simulink model "ctrlAllocMatrix_th"  (R2018b)
settings: Solver=FixedStepDiscrete  StartTime=0.0  StopTime=timeVec(end)  FixedStep=1  RelTol=1e-3
values from neighbouring files (symbols this model uses):
  angVelBdy = [0 0 0]*pi/180    [ctrlAllocMatrix_ts.m]
  velCMBdy = [0 0 0]    [ctrlAllocMatrix_ts.m]
undefined symbols (not defined in the file or in its folder): vhcl
libraries: fluidDynamicSurface_cl x4, ctrlAllocMatrix_cl x1
settings Model: Creator=mcobb  LastModifiedBy=mcobb

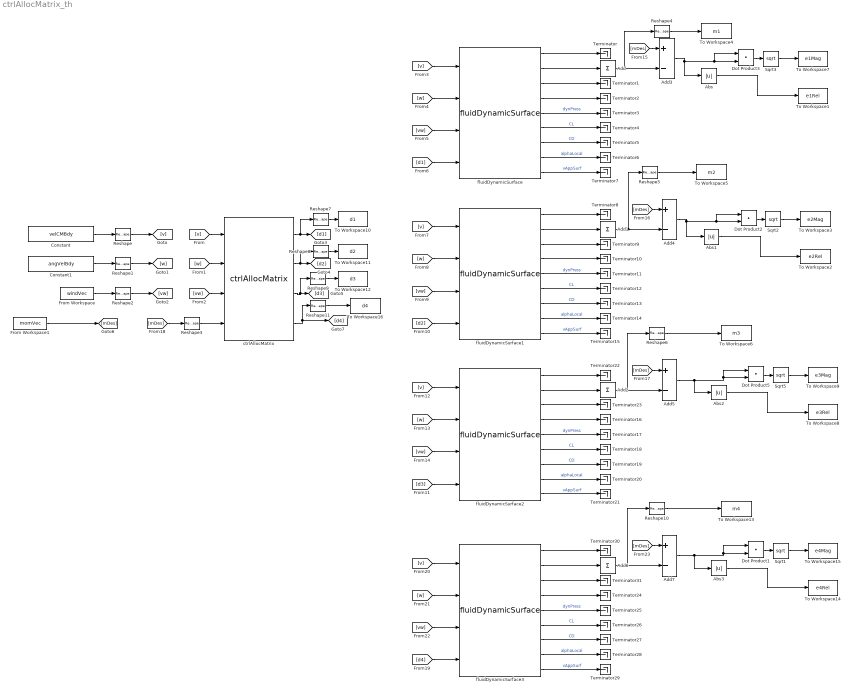
== system ctrlAllocMatrix_th ==
  Abs{,1..3} (4 alike) : Abs
  Add{,1..2,6} (4 alike) : Sum  Inputs=1  CollapseMode=Specified dimension  CollapseDim=2
  Add{3..5,7} (4 alike) : Sum  Inputs=+-
  Constant : Constant  Value=velCMBdy
  Constant1 : Constant  Value=angVelBdy
  Dot Product{1..3,5} (4 alike) : DotProduct  InputSameDT=on  OutDataTypeStr=Inherit: Inherit via internal rule
  From Workspace : FromWorkspace  VariableName=windVec  SampleTime=0
  From Workspace1 : FromWorkspace  VariableName=momVec  SampleTime=0
  Reshape{,1..3} (4 alike) : Reshape  OutputDimensionality=Column vector (2-D)
  Reshape{4..11} (8 alike) : Reshape
  Sqrt{1..3,5} (4 alike) : Sqrt  SaturateOnIntegerOverflow=on
  Terminator{,1..31} (32 alike) : Terminator
  To Workspace1 : ToWorkspace  VariableName=e1Rel  SaveFormat=Timeseries  SampleTime=-1
  To Workspace10 : ToWorkspace  VariableName=d1  SaveFormat=Timeseries  SampleTime=-1
  To Workspace11 : ToWorkspace  VariableName=d2  SaveFormat=Timeseries  SampleTime=-1
  To Workspace12 : ToWorkspace  VariableName=d3  SaveFormat=Timeseries  SampleTime=-1
  To Workspace13 : ToWorkspace  VariableName=m4  SaveFormat=Timeseries  SampleTime=-1
  To Workspace14 : ToWorkspace  VariableName=e4Rel  SaveFormat=Timeseries  SampleTime=-1
  To Workspace15 : ToWorkspace  VariableName=e4Mag  SaveFormat=Timeseries  SampleTime=-1
  To Workspace16 : ToWorkspace  VariableName=d4  SaveFormat=Timeseries  SampleTime=-1
  To Workspace2 : ToWorkspace  VariableName=e2Rel  SaveFormat=Timeseries  SampleTime=-1
  To Workspace3 : ToWorkspace  VariableName=e2Mag  SaveFormat=Timeseries  SampleTime=-1
  To Workspace4 : ToWorkspace  VariableName=m1  SaveFormat=Timeseries  SampleTime=-1
  To Workspace5 : ToWorkspace  VariableName=m2  SaveFormat=Timeseries  SampleTime=-1
  To Workspace6 : ToWorkspace  VariableName=m3  SaveFormat=Timeseries  SampleTime=-1
  To Workspace7 : ToWorkspace  VariableName=e1Mag  SaveFormat=Timeseries  SampleTime=-1
  To Workspace8 : ToWorkspace  VariableName=e3Rel  SaveFormat=Timeseries  SampleTime=-1
  To Workspace9 : ToWorkspace  VariableName=e3Mag  SaveFormat=Timeseries  SampleTime=-1
  ctrlAllocMatrix : ctrlAllocMatrix_cl/ctrlAllocMatrix  aeroStruct=vhcl.struct('OCT.aeroSurf')  fluidDensity=1000  ctrlUpMax=30  ctrlDnMax=-30
  fluidDynamicSurface{,1..3} (4 alike) : fluidDynamicSurface_cl/fluidDynamicSurface  aeroStruct=vhcl.struct('OCT.aeroSurf')  fluidDensity=1000
  wires:
  Constant/1 -> Reshape/1
  Constant1/1 -> Reshape1/1
  From Workspace/1 -> Reshape2/1
  From Workspace1/1 -> [mDes]
  Reshape3/1 -> ctrlAllocMatrix/4
  Reshape/1 -> [v]
  [v] -> ctrlAllocMatrix/1
  [w] -> ctrlAllocMatrix/2
  Reshape1/1 -> [w]
  Reshape2/1 -> [vw]
  [vw] -> ctrlAllocMatrix/3
  [v] -> fluidDynamicSurface/1
  [w] -> fluidDynamicSurface/2
  [vw] -> fluidDynamicSurface/3
  fluidDynamicSurface/1 -> Terminator/1
  fluidDynamicSurface/2 -> Add/1
  fluidDynamicSurface/3 -> Terminator1/1
  fluidDynamicSurface/4 -> Terminator2/1
  fluidDynamicSurface/5 -> Terminator3/1  "dynPress"
  fluidDynamicSurface/6 -> Terminator4/1  "CL"
  fluidDynamicSurface/7 -> Terminator5/1  "CD"
  fluidDynamicSurface/8 -> Terminator6/1  "alphaLocal"
  fluidDynamicSurface/9 -> Terminator7/1  "vAppSurf"
  Add/1 -> Reshape4/1, Add3/2
  ctrlAllocMatrix/1 -> Reshape7/1, [d1]
  ctrlAllocMatrix/2 -> Reshape8/1, [d2]
  ctrlAllocMatrix/3 -> Reshape9/1, [d3]
  [d1] -> fluidDynamicSurface/4
  [d2] -> fluidDynamicSurface1/4
  fluidDynamicSurface1/9 -> Terminator15/1  "vAppSurf"
  fluidDynamicSurface1/8 -> Terminator14/1  "alphaLocal"
  fluidDynamicSurface1/7 -> Terminator13/1  "CD"
  fluidDynamicSurface1/6 -> Terminator12/1  "CL"
  fluidDynamicSurface1/5 -> Terminator11/1  "dynPress"
  fluidDynamicSurface1/4 -> Terminator10/1
  fluidDynamicSurface1/3 -> Terminator9/1
  fluidDynamicSurface1/2 -> Add1/1
  fluidDynamicSurface1/1 -> Terminator8/1
  [vw] -> fluidDynamicSurface1/3
  [w] -> fluidDynamicSurface1/2
  [v] -> fluidDynamicSurface1/1
  [v] -> fluidDynamicSurface2/1
  [w] -> fluidDynamicSurface2/2
  [vw] -> fluidDynamicSurface2/3
  fluidDynamicSurface2/1 -> Terminator22/1
  fluidDynamicSurface2/2 -> Add2/1
  fluidDynamicSurface2/3 -> Terminator23/1
  fluidDynamicSurface2/4 -> Terminator16/1
  fluidDynamicSurface2/5 -> Terminator17/1  "dynPress"
  fluidDynamicSurface2/6 -> Terminator18/1  "CL"
  fluidDynamicSurface2/7 -> Terminator19/1  "CD"
  fluidDynamicSurface2/8 -> Terminator20/1  "alphaLocal"
  fluidDynamicSurface2/9 -> Terminator21/1  "vAppSurf"
  [d3] -> fluidDynamicSurface2/4
  [mDes] -> Add3/1
  Add3/1 -> Dot Product3/1, Dot Product3/2, Abs/1
  [mDes] -> Add4/1
  Add1/1 -> Reshape5/1, Add4/2
  Add2/1 -> Reshape6/1, Add5/2
  [mDes] -> Add5/1
  [mDes] -> Reshape3/1
  Abs/1 -> To Workspace1/1
  Reshape4/1 -> To Workspace4/1
  Reshape5/1 -> To Workspace5/1
  Reshape6/1 -> To Workspace6/1
  Dot Product3/1 -> Sqrt3/1
  Sqrt3/1 -> To Workspace7/1
  Sqrt2/1 -> To Workspace3/1
  Dot Product2/1 -> Sqrt2/1
  Abs1/1 -> To Workspace2/1
  Add4/1 -> Abs1/1, Dot Product2/2, Dot Product2/1
  Add5/1 -> Dot Product5/1, Dot Product5/2, Abs2/1
  Abs2/1 -> To Workspace8/1
  Dot Product5/1 -> Sqrt5/1
  Sqrt5/1 -> To Workspace9/1
  Reshape7/1 -> To Workspace10/1
  Reshape8/1 -> To Workspace11/1
  Reshape9/1 -> To Workspace12/1
  Sqrt1/1 -> To Workspace15/1
  Dot Product1/1 -> Sqrt1/1
  Abs3/1 -> To Workspace14/1
  Add7/1 -> Abs3/1, Dot Product1/2, Dot Product1/1
  Reshape10/1 -> To Workspace13/1
  [mDes] -> Add7/1
  Add6/1 -> Add7/2, Reshape10/1
  [d4] -> fluidDynamicSurface3/4
  fluidDynamicSurface3/9 -> Terminator29/1  "vAppSurf"
  fluidDynamicSurface3/8 -> Terminator28/1  "alphaLocal"
  fluidDynamicSurface3/7 -> Terminator27/1  "CD"
  fluidDynamicSurface3/6 -> Terminator26/1  "CL"
  fluidDynamicSurface3/5 -> Terminator25/1  "dynPress"
  fluidDynamicSurface3/4 -> Terminator24/1
  fluidDynamicSurface3/3 -> Terminator31/1
  fluidDynamicSurface3/2 -> Add6/1
  fluidDynamicSurface3/1 -> Terminator30/1
  [vw] -> fluidDynamicSurface3/3
  [w] -> fluidDynamicSurface3/2
  [v] -> fluidDynamicSurface3/1
  ctrlAllocMatrix/4 -> [d4], Reshape11/1
  Reshape11/1 -> To Workspace16/1
